simulink model "untitled09"  (Simulink 7.3)
settings: Solver=ode45  StartTime=0.0  StopTime=10.0  RelTol=1e-3
undefined symbols (not defined in the file or in its folder): i
libraries: commchan3 x1, commrandsrc2 x1, commdigbbndam3 x1, dspspect3 x1
settings Model: Creator=YMTS0534  LastModifiedBy=YMTS0534

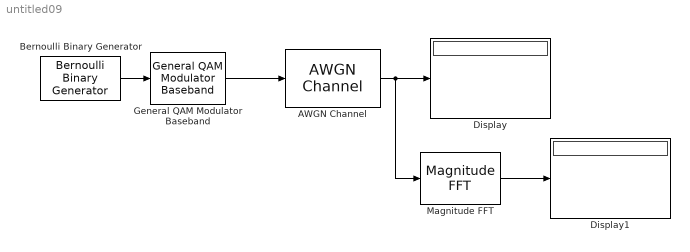
== system untitled09 ==
  AWGN Channel : commchan3/AWGN Channel  SystemSampleTime=-1  seed=67  noiseMode="Signal to noise ratio  (SNR)"  EbNodB=10  EsNodB=10  SNRdB=10  bitsPerSym=1  Ps=1  Tsym=1  variance=1
  Bernoulli Binary Generator : commrandsrc2/Bernoulli Binary Generator  DialogController=commDDGCreate  DialogControllerArgs=DataTag0  SystemSampleTime=-1  P=0.5  seed=61  Ts=1  frameBased=off  sampPerFrame=1  orient=off  outDataType=double
  Display : Display
  Display1 : Display
  General QAM Modulator Baseband : commdigbbndam3/General QAM Modulator Baseband  DialogController=commDDGCreate  DialogControllerArgs=DataTag1  SigCon=[exp(2*pi*i*[0:7]/8)]  outDtype=double  outWordLen=16  outUDDataType=sfix(16)  outFracLenMode=Best precision  outFracLen=15
  Magnitude FFT : dspspect3/Magnitude FFT  SystemSampleTime=-1  mag_or_magsq=Magnitude squared  fftLenInherit=off  fftsize=256
  wires:
  Bernoulli Binary Generator/1 -> General QAM Modulator Baseband/1
  General QAM Modulator Baseband/1 -> AWGN Channel/1
  AWGN Channel/1 -> Display/1, Magnitude FFT/1
  Magnitude FFT/1 -> Display1/1
